simulink model "fmu_steady_timesteps"  (R2023b)
settings: Solver=FixedStepAuto  StartTime=0.0  StopTime=10  FixedStep=0.01  RelTol=1e-3
undefined symbols (not defined in the file or in its folder): egl
settings Model: Creator=pcelel  LastModifiedBy=stefan.rudolph
settings DataIOCC: SaveFinalState=on  SaveFormat=Array  LoggingFileName=out1.mat

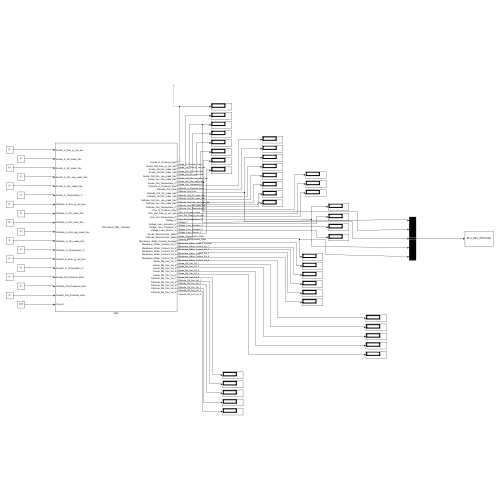
[thumbnail: Simulink's stored preview of the top-level diagram]
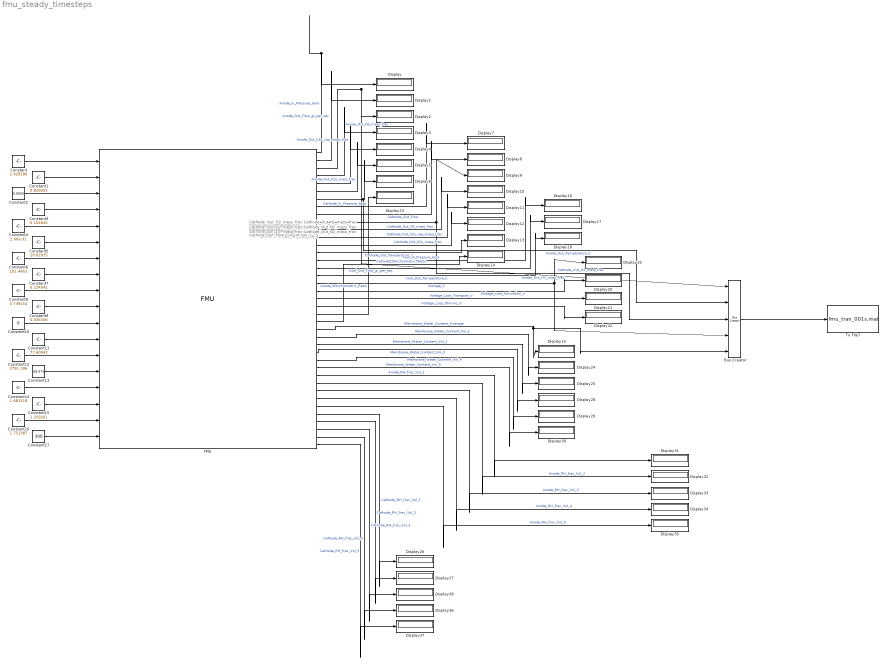
== system fmu_steady_timesteps ==
  note: Cathode_RH_frac_Vol_1
  note: Anode_RH_frac_Vol_1
  note: Anode_RH_frac_Vol_1
  note: Anode_RH_frac_Vol_1
  note: Anode_RH_frac_Vol_1
  note: Anode_RH_frac_Vol_1
  note: Anode_RH_frac_Vol_1
  note: Anode_RH_frac_Vol_1
  note: Membrane_Water_Content_Vol_1
  note: Voltage_Loss_Transport_V
  note: Cool_Out_Flow_gr_per_sec
  note: Cathode_Out_O2_mass_frac
      |
      | Cathode_Out_N2_mass_frac
  note: Cathode_Out_O2_mass_frac
      |
      | Cathode_Out_N2_mass_frac
  note: Cathode_Out_O2_mass_frac
      |
      | Cathode_Out_N2_mass_frac
  note: Cathode_Out_O2_mass_frac
      |
      | Cathode_Out_N2_mass_frac
  note: Cathode_Out_O2_mass_frac
      |
      | Cathode_Out_N2_mass_frac
  note: Cathode_Out_Flow
  note: Cathode_Out_Flow
  note: Cathode_Out_Flow
  Bus Creator : BusCreator  Inputs=5
  Constant : Constant  Value=1.928186
  Constant1 : Constant  Value=0.826055
  Constant10 : Constant  Value=0
  Constant11 : Constant  Value=77.60942
  Constant12 : Constant  Value=2791.186
  Constant13 : Constant  Value=68.073
  Constant14 : Constant  Value=1.681518
  Constant15 : Constant  Value=1.259201
  Constant16 : Constant  Value=1.751387
  Constant17 : Constant  Value=300
  Constant2 : Constant  Value=0.0693
  Constant3 : Constant  Value=0.104645
  Constant4 : Constant  Value=2.66e-32
  Constant5 : Constant  Value=29.82035
  Constant6 : Constant  Value=101.4453
  Constant7 : Constant  Value=0.224541
  Constant8 : Constant  Value=0.739154
  Constant9 : Constant  Value=0.036306
  Display{,1..38} (39 alike) : Display
  FMU : FMU  FMUName=P02_Stack_FMU_Transient.fmu  FMUDebugLogging=on  FMUMode=CoSimulation  FMUCachedDialogLayout="{\"Geometry\":[2660,489,1052,738],\"ParameterColumnsWidthConfig\":\"{\\\"columns\\\":[{\\\"name\\\":\\\"Parameter\\\",\\\"width\\\":269},{\\\"name\\\":\\\"Value\\\",\\\"width\\\":240},{\\\"name\\\":\\\"Unit\\\",\\\"width\\\":232},{\\\"name\\\":\\\"Description\\\",\\\"width\\\":274}]}\",\"InputColumnsWidthConfig\":\"{\\\"columns\\\":[{\\\"name\\\":\\\"Name\\\",\\\"width\\\":234},{\\\"name\\\":\\\"Visibility\\\",\\\"width\\\":60},{\\\"name\\\":\\\"Start\\\",\\\"width\\\":226},{\\\"name\\\":\\\"Unit\\\",\\\"width\\\":222},{\\\"name\\\":\\\"Type Object\\\",\\\"width\\\":269}]}\",\"OutputColumnsWidthConfig\":\"{\\\"columns\\\":[{\\\"name\\\":\\\"Name\\\",\\\"width\\\":234},{\\\"name\\\":\\\"Visibility\\\",\\\"width\\\":60},{\\\"name\\\":\\\"Start\\\",\\\"width\\\":226},{\\\"name\\\":\\\"Unit\\\",\\\"width\\\":222},{\\\"name\\\":\\\"Type Object\\\",\\\"width\\\":269}]}\"}"  Anode_Inlet_Diameter_mm=20  Anode_Outlet_Diameter_mm=20  Cathode_Inlet_Diameter_mm=60  Cathode_Outlet_Diameter_mm=60  Discretization_length_mm=100  Coolant_Inlet_Diameter=50  Coolant_Outlet_Diameter=50  Anode_Initial_Pressure_bara=1  Anode_Initial_Temperature_C=40  Anode_Initial_H2_Vol_Frac=0.9  Anode_Initial_RH_Frac=0.5  Cathode_Initial_Pressure_bara=1  Cathode_Initial_Temperature_C=50  Cathode_Initial_RH_Frac=0.5  Coolant_Initial_Temperature_C=68.238304  Coolant_Initial_Pressure_bara=1  Stack_Initial_Temperature_C=70  Coolant_fluid=egl-5050  mask(P02_Stack_FMU_Transient [Co-Simulation, v2.0]){}
      mask Display:
      | disp('P02_Stack_FMU_Transient');
      | port_label('output',1,'Anode_In_Pressure_bara');
      | port_label('output',2,'Anode_Out_Flow_gr_per_sec');
      | port_label('output',3,'Anode_Out_H2_mass_frac');
      | port_label('output',4,'Anode_Out_N2_mass_frac');
      | port_label('output',5,'Anode_Out_h2o_vap_mass_frac');
      | port_label('output',6,'Anode_Out_h2o_mass_frac');
      | port_label('output',7,'Anode_Out_Temperature_C');
      | port_label('output',8,'Cathode_In_Pressure_bara');
      | port_label('output',9,'Cathode_Out_Flow');
      | port_label('output',10,'Cathode_Out_O2_mass_frac');
      | port_label('output',11,'Cathode_Out_N2_mass_frac');
      | port_label('output',12,'Cathode_Out_h2o_vap_mass_frac');
      | port_label('output',13,'Cathode_Out_h2o_mass_frac');
      | port_label('output',14,'Cathode_Out_Temperature_C');
      | port_label('output',15,'Cool_In_Pressure_bara');
      | port_label('output',16,'Cool_Out_Flow_gr_per_sec');
      | port_label('output',17,'Cool_Out_Temperature_C');
      | port_label('output',18,'Voltage_V');
      | port_label('output',19,'Voltage_Loss_Activation_V');
      | port_label('output',20,'Voltage_Loss_Transport_V');
      | port_label('output',21,'Voltage_Loss_Ohmnic_V');
      | port_label('output',22,'Anode_Stoichiometric_Ratio');
      | port_label('output',23,'Cathode_Stoichiometric_Ratio');
      | port_label('output',24,'Membrane_Water_Content_Average');
      | port_label('output',25,'Membrane_Water_Content_Vol_1');
      | port_label('output',26,'Membrane_Water_Content_Vol_2');
      | port_label('output',27,'Membrane_Water_Content_Vol_3');
      | port_label('output',28,'Membrane_Water_Content_Vol_4');
      | port_label('output',29,'Membrane_Water_Content_Vol_5');
      | port_label('output',30,'Anode_RH_frac_Vol_1');
      | port_label('output',31,'Anode_RH_frac_Vol_2');
      | port_label('output',32,'Anode_RH_frac_Vol_3');
      | port_label('output',33,'Anode_RH_frac_Vol_4');
      | port_label('output',34,'Anode_RH_frac_Vol_5');
      | port_label('output',35,'Cathode_RH_frac_Vol_1');
      | port_label('output',36,'Cathode_RH_frac_Vol_2');
      | port_label('output',37,'Cathode_RH_frac_Vol_3');
      | port_label('output',38,'Cathode_RH_frac_Vol_4');
      | port_label('output',39,'Cathode_RH_frac_Vol_5');
      | port_label('input',1,'Anode_In_flow_gr_per_sec');
      | port_label('input',2,'Anode_In_H2_mass_frac');
      | port_label('input',3,'Anode_In_N2_mass_frac');
      | port_label('input',4,'Anode_In_h2o_vap_mass_frac');
      | port_label('input',5,'Anode_In_h2o_mass_frac');
      | port_label('input',6,'Anode_In_Temperature_C');
      | port_label('input',7,'Cathode_In_flow_gr_per_sec');
      | port_label('input',8,'Cathode_In_O2_mass_frac');
      | port_label('input',9,'Cathode_In_N2_mass_frac');
      | port_label('input',10,'Cathode_In_h2o_vap_mass_frac');
      | port_label('input',11,'Cathode_In_h2o_mass_frac');
      | port_label('input',12,'Cathode_In_Temperature_C');
      | port_label('input',13,'Coolant_In_Flow_gr_per_sec');
      | port_label('input',14,'Coolant_In_Temperature_C');
      | port_label('input',15,'Anode_Out_Pressure_bara');
      | port_label('input',16,'Cathode_Out_Pressure_bara');
      | port_label('input',17,'Coolant_Out_Pressure_bara');
      | port_label('input',18,'Current');
  To File7 : ToFile  Filename=fmu_tran_001s.mat  MatrixName=fmu_tran_001s
  wires:
  Constant/1 -> FMU/1
  Constant4/1 -> FMU/5
  Constant2/1 -> FMU/3
  Constant1/1 -> FMU/2
  Constant3/1 -> FMU/4
  Constant5/1 -> FMU/6
  Constant6/1 -> FMU/7
  Constant7/1 -> FMU/8
  Constant8/1 -> FMU/9
  Constant9/1 -> FMU/10
  Constant10/1 -> FMU/11
  Constant11/1 -> FMU/12
  Constant12/1 -> FMU/13
  Constant13/1 -> FMU/14
  Constant14/1 -> FMU/15
  Constant15/1 -> FMU/16
  Constant16/1 -> FMU/17
  Constant17/1 -> FMU/18
  FMU/1 -> Display/1  "Anode_In_Pressure_bara"
  FMU/2 -> Display1/1  "Anode_Out_Flow_gr_per_sec"
  FMU/3 -> Bus Creator/1, Display2/1  "Anode_Out_H2_mass_frac"
  FMU/5 -> Display4/1  "Anode_Out_h2o_vap_mass_frac"
  FMU/6 -> Display5/1  "Anode_Out_h2o_mass_frac"
  FMU/4 -> Display3/1  "Anode_Out_N2_mass_frac"
  FMU/8 -> Display7/1  "Cathode_In_Pressure_bara"
  FMU/9 -> Display8/1  "Cathode_Out_Flow"
  FMU/7 -> Bus Creator/2, Display6/1  "Anode_Out_Temperature_C"
  FMU/11 -> Display10/1  "Cathode_Out_N2_mass_frac"
  FMU/12 -> Display11/1  "Cathode_Out_h2o_vap_mass_frac"
  FMU/10 -> Bus Creator/3, Display9/1  "Cathode_Out_O2_mass_frac"
  FMU/20 -> Display21/1  "Voltage_Loss_Transport_V"
  FMU/21 -> Display22/1  "Voltage_Loss_Ohmnic_V"
  FMU/19 -> Display20/1  "Voltage_Loss_Activation_V"
  FMU/14 -> Display13/1  "Cathode_Out_Temperature_C"
  FMU/22 -> Display23/1  "Anode_Stoichiometric_Ratio"
  FMU/23 -> Display14/1  "Cathode_Stoichiometric_Ratio"
  FMU/24 -> Bus Creator/5, Display15/1  "Membrane_Water_Content_Average"
  FMU/13 -> Display12/1  "Cathode_Out_h2o_mass_frac"
  FMU/17 -> Display18/1  "Cool_Out_Temperature_C"
  FMU/15 -> Display16/1  "Cool_In_Pressure_bara"
  FMU/18 -> Display19/1, Bus Creator/4  "Voltage_V"
  FMU/16 -> Display17/1  "Cool_Out_Flow_gr_per_sec"
  FMU/32 -> Display33/1  "Anode_RH_frac_Vol_3"
  FMU/33 -> Display34/1  "Anode_RH_frac_Vol_4"
  FMU/31 -> Display32/1  "Anode_RH_frac_Vol_2"
  FMU/26 -> Display25/1  "Membrane_Water_Content_Vol_2"
  FMU/34 -> Display35/1  "Anode_RH_frac_Vol_5"
  FMU/35 -> Display26/1  "Cathode_RH_frac_Vol_1"
  FMU/36 -> Display27/1  "Cathode_RH_frac_Vol_2"
  FMU/25 -> Display24/1  "Membrane_Water_Content_Vol_1"
  FMU/29 -> Display30/1  "Membrane_Water_Content_Vol_5"
  FMU/27 -> Display28/1  "Membrane_Water_Content_Vol_3"
  FMU/30 -> Display31/1  "Anode_RH_frac_Vol_1"
  FMU/28 -> Display29/1  "Membrane_Water_Content_Vol_4"
  FMU/37 -> Display38/1  "Cathode_RH_frac_Vol_3"
  FMU/38 -> Display36/1  "Cathode_RH_frac_Vol_4"
  FMU/39 -> Display37/1  "Cathode_RH_frac_Vol_5"
  Bus Creator/1 -> To File7/1
